simulink model "MGTestSystem_4bus"  (R2021b)
settings: Solver=VariableStepAuto  StartTime=0.0  StopTime=4  RelTol=1e-3
PreLoadFcn:
  | addpath Icons
  | addpath Util
InitFcn:
  | clc
  | %clear all
  | 
  | nDER = 4;
  | xssum = zeros(nDER*2,1);
  | save XSSUM xssum
  | 
  | Ts_Control=1e-4;       % local control time step
  | Ts_Simulation=5e-5;   %simulation time step
  | Ts_Power=5e-5;   % measurement time step
  | Tdisc=0.8;     % time setting for disconnecting from the main grid
  | 
  | Iref = 0.3;  % in p.u.
  | Iqref = 0;  % in p.u.
  | 
  | Ts_secondary =3e-2;   %  secondary control time step
  | %Ts_PMU = 1/60;
  | 
  | ft2km=3.0480e-04;
  | 
  | KPdroop=3.4e-4;
  | KQdroop=1e-3/1;
  | KPdroop2=4.5e-4;
  | KQdroop2=1.5e-3/1;
  | 
  | %KWinvdroop = 20.0;
  | %KVinvdroop = 16.7;
  | %KWinvdroop = 0.05;
  | %KVinvdroop = 0.08;
  | 
  | KWinvdroop = 1/(2*pi*KPdroop);
  | KVinvdroop = 1/(2*pi*KQdroop)
  | KWinvdroop2 = 1/(2*pi*KPdroop2);
  | KVinvdroop2 = 1/(2*pi*KQdroop2)
  | %KVinvdroop = 1/(KQdroop);
  | %KVinvdroop2 = 1/(KQdroop2);
  | %KWinvdroop = 1/(KPdroop);
  | %KWinvdroop2 = 1/(KPdroop2);
  | 
  | droopv1=1/KVinvdroop
  | droopv2=1/KVinvdroop2
  | 
  | 
  | 
  | 
  | wfilter = 35;
  | Rv=0.0;
  | Lv=0e-3;
  | 
  | div=1;
  | 
  | 
  | Kpac=0.1/1;
  | Kiac=420/1;
  | Kpaci=15/div;
  | Kiaci=2e3/div;
  | Kpac2=0.05/1;
  | Kiac2=390/1;
  | Kpaci2=15/div;
  | Kiaci2=1.6e3/div;
  | 
  | 
  | Kpac=0.5/div;
  | Kiac=53/div;
  | Kpaci=45/div;
  | Kiaci=450/div;
  | Kpac2=0.5/div;
  | Kiac2=34/div;
  | Kpaci2=35/div;
  | Kiaci2=353/div;
  | 
  | 
  | Kpac=0.1256/div;
  | Kiac=950/div;
  | Kpaci=20.6/div;
  | Kiaci=1522.7/div;
  | Kpac2=0.1256/div;
  | Kiac2=591/div;
  | Kpaci2=20.6/div;
  | Kiaci2=1522.7/div;
  | 
  | 
  | Kpac=0.5;  % K_I for voltage PI
  | Kiac=523;  % K_I for voltage PI
  | Kpac2=0.5; % K_P for voltage PI 2
  | Kiac2=523; % K_I for voltage PI 2
  | Kpaci=0.3;  % K_P for current PI
  | Kiaci=635;   % K_I for current PI
  | Kpaci2=0.3;  % K_P for current PI 2
  | Kiaci2=635;  % K_I for current PI 2
  | 
  | 
  | k=1;
  | 
  | Pvscr = 30e3;
  | VDC = 950;
  | 
  | %PDERS1 = 12e3;
  | %QDERS1 = 6e3;
  | %PDERS2 = 12e3;
  | %QDERS2 = 6e3;
  | %PDERS3 = 12e3;
  | %QDERS3 = 6e3;
  | %PDERS4 = 12e3;
  | %QDERS4= 6e3;
  | 
  | %[params,indctor] = initfuncv1();
undefined symbols (not defined in the file or in its folder): D1, Delta, Ion, Lithium
libraries: spsStairGeneratorLib x24, spsThreePhaseSeriesRLCBranchLib x24, powerlib_extras x23, spsSeriesRLCBranchLib x20, spsThreePhaseVIMeasurementLib x18, slpidlib x18, spsThreePhaseBreakerLib x15, spsRMSLib x10, spsThreePhaseSeriesRLCLoadLib x8, spsVoltageMeasurementLib x8, spsPMUPLLBasedPositiveSequenceLib x6, spsPowerLib x5
(part 1 of 7)
settings Model: Creator=gongx  LastModifiedBy=gongx
settings SolverCC: ZeroCrossAlgorithm=Adaptive
settings DataIOCC: SaveOutput=off  SignalLogging=off  DSMLogging=off  ReturnWorkspaceOutputs=off
settings DebuggingCC: MaskedZcDiagnostic=none  IgnoredZcDiagnostic=none  UnderSpecifiedDimensionMsg=warning

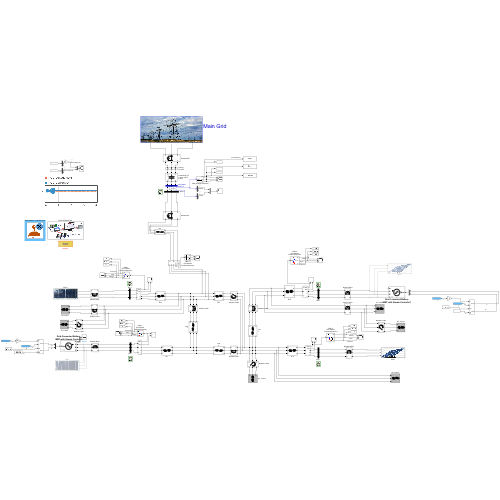
[thumbnail: Simulink's stored preview of the top-level diagram]
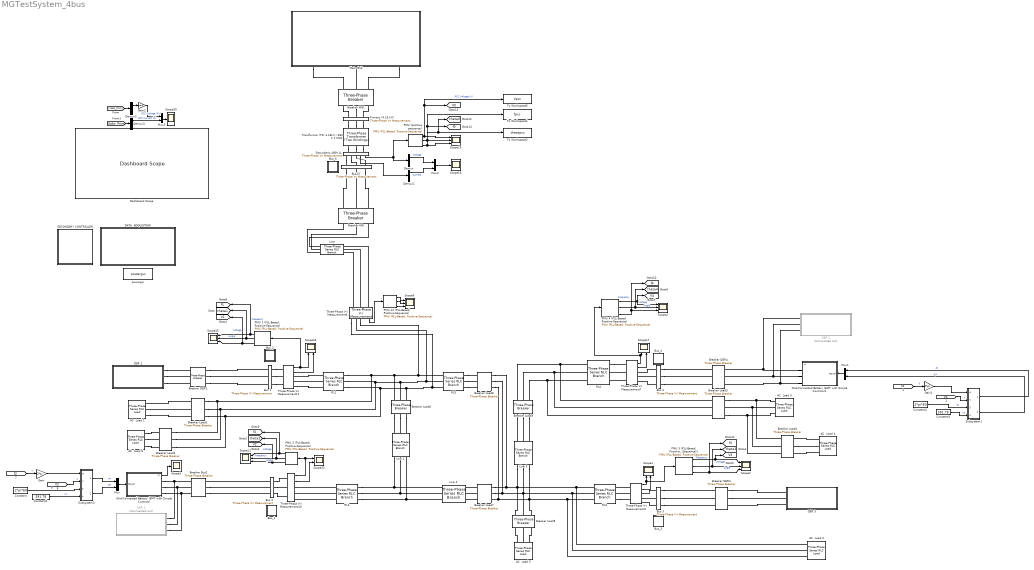
== system MGTestSystem_4bus ==
  " Bus13" : spsThreePhaseVIMeasurementLib/Three-Phase V-I Measurement  VoltageMeasurement=phase-to-ground  SetLabelV=on  LabelV=Vabc_LL_Bus13  Vpu=off  VpuLL=off  CurrentMeasurement=yes  SetLabelI=on  LabelI=Iabc_LL_Bus13  Ipu=off  Pbase=100e6  Vbase=500e3  OutputType=Complex  PhasorSimulation=off  PSBequivalent=0
  AC  Load 1 : spsThreePhaseSeriesRLCLoadLib/Three-Phase Series RLC Load  LConnTagsString=A|B|C  Configuration=Y (grounded)  NominalVoltage=480  Vabc=[1e3 1e3 1e3]  Vabcp=[1e3 1e3 1e3]  NominalFrequency=60  UnbalancedPower=off  ActivePower=20e3  InductivePower=9e3  CapacitivePower=0  Pabc=[10e3 9e3 11e3]  QLabc=[100 90 110]  QCabc=[100 90 110]  Pabcp=[10e3 9e3 11e3]  QLabcp=[100 90 110]  QCabcp=[100 90 110]  Measurements=None  LoadType=constant PQ
  AC  Load 2 : spsThreePhaseSeriesRLCLoadLib/Three-Phase Series RLC Load  LConnTagsString=A|B|C  Configuration=Y (grounded)  NominalVoltage=480  Vabc=[1e3 1e3 1e3]  Vabcp=[1e3 1e3 1e3]  NominalFrequency=60  UnbalancedPower=off  ActivePower=16e3  InductivePower=9e3  CapacitivePower=0  Pabc=[10e3 9e3 11e3]  QLabc=[100 90 110]  QCabc=[100 90 110]  Pabcp=[10e3 9e3 11e3]  QLabcp=[100 90 110]  QCabcp=[100 90 110]  Measurements=None  LoadType=constant PQ
  AC  Load 3 : spsThreePhaseSeriesRLCLoadLib/Three-Phase Series RLC Load  LConnTagsString=A|B|C  Configuration=Y (grounded)  NominalVoltage=480  Vabc=[1e3 1e3 1e3]  Vabcp=[1e3 1e3 1e3]  NominalFrequency=60  UnbalancedPower=off  ActivePower=12e3  InductivePower=6e3  CapacitivePower=0  Pabc=[10e3 9e3 11e3]  QLabc=[100 90 110]  QCabc=[100 90 110]  Pabcp=[10e3 9e3 11e3]  QLabcp=[100 90 110]  QCabcp=[100 90 110]  Measurements=None  LoadType=constant PQ
  AC  Load 4 : spsThreePhaseSeriesRLCLoadLib/Three-Phase Series RLC Load  LConnTagsString=A|B|C  Configuration=Y (grounded)  NominalVoltage=480  Vabc=[1e3 1e3 1e3]  Vabcp=[1e3 1e3 1e3]  NominalFrequency=60  UnbalancedPower=off  ActivePower=10e3  InductivePower=6e3  CapacitivePower=0  Pabc=[10e3 9e3 11e3]  QLabc=[100 90 110]  QCabc=[100 90 110]  Pabcp=[10e3 9e3 11e3]  QLabcp=[100 90 110]  QCabcp=[100 90 110]  Measurements=None  LoadType=constant PQ
  AC  Load 5 : spsThreePhaseSeriesRLCLoadLib/Three-Phase Series RLC Load  LConnTagsString=A|B|C  Configuration=Y (grounded)  NominalVoltage=480  Vabc=[1e3 1e3 1e3]  Vabcp=[1e3 1e3 1e3]  NominalFrequency=60  UnbalancedPower=off  ActivePower=60e3  InductivePower=30e3  CapacitivePower=0  Pabc=[10e3 9e3 11e3]  QLabc=[100 90 110]  QCabc=[100 90 110]  Pabcp=[10e3 9e3 11e3]  QLabcp=[100 90 110]  QCabcp=[100 90 110]  Measurements=None  LoadType=constant PQ
  AC  Load 6 : spsThreePhaseSeriesRLCLoadLib/Three-Phase Series RLC Load  LConnTagsString=A|B|C  Configuration=Y (grounded)  NominalVoltage=480  Vabc=[1e3 1e3 1e3]  Vabcp=[1e3 1e3 1e3]  NominalFrequency=60  UnbalancedPower=off  ActivePower=50e3  InductivePower=30e3  CapacitivePower=0  Pabc=[10e3 9e3 11e3]  QLabc=[100 90 110]  QCabc=[100 90 110]  Pabcp=[10e3 9e3 11e3]  QLabcp=[100 90 110]  QCabcp=[100 90 110]  Measurements=None  LoadType=constant PQ
  "Breaker Bus2 " : spsThreePhaseBreakerLib/Three-Phase Breaker  InitialState=closed  SwitchA=on  SwitchB=on  SwitchC=on  SwitchTimes=[113.3 200]  External=off  BreakerResistance=0.001  SnubberResistance=1e6  SnubberCapacitance=inf  Measurements=None
  Breaker DER1 : spsThreePhaseBreakerLib/Three-Phase Breaker  InitialState=closed  SwitchA=on  SwitchB=on  SwitchC=on  SwitchTimes="[10.9  314]"  External=off  BreakerResistance=0.001  SnubberResistance=1e6  SnubberCapacitance=inf  Measurements=None
  Breaker DER3 : spsThreePhaseBreakerLib/Three-Phase Breaker  InitialState=closed  SwitchA=on  SwitchB=on  SwitchC=on  SwitchTimes="[112.7  123.4]"  External=off  BreakerResistance=0.001  SnubberResistance=1e6  SnubberCapacitance=inf  Measurements=None
  Breaker DER4 : spsThreePhaseBreakerLib/Three-Phase Breaker  InitialState=closed  SwitchA=on  SwitchB=on  SwitchC=on  SwitchTimes="[112.7  300.4]"  External=off  BreakerResistance=0.001  SnubberResistance=1e6  SnubberCapacitance=inf  Measurements=None
  Breaker Load1 : spsThreePhaseBreakerLib/Three-Phase Breaker  InitialState=closed  SwitchA=on  SwitchB=on  SwitchC=on  SwitchTimes="[111.8  113.3]"  External=off  BreakerResistance=0.001  SnubberResistance=1e6  SnubberCapacitance=inf  Measurements=None
  Breaker Load2 : spsThreePhaseBreakerLib/Three-Phase Breaker  InitialState=open  SwitchA=on  SwitchB=on  SwitchC=on  SwitchTimes="[10.9  112.3]"  External=off  BreakerResistance=0.001  SnubberResistance=1e6  SnubberCapacitance=inf  Measurements=None
  Breaker Load3 : spsThreePhaseBreakerLib/Three-Phase Breaker  InitialState=closed  SwitchA=on  SwitchB=on  SwitchC=on  SwitchTimes="[112.2  113.3]"  External=off  BreakerResistance=0.001  SnubberResistance=1e6  SnubberCapacitance=inf  Measurements=None
  Breaker Load4 : spsThreePhaseBreakerLib/Three-Phase Breaker  InitialState=open  SwitchA=on  SwitchB=on  SwitchC=on  SwitchTimes="[13.0  120.6]"  External=off  BreakerResistance=0.001  SnubberResistance=1e6  SnubberCapacitance=inf  Measurements=None
  Breaker Load5 : spsThreePhaseBreakerLib/Three-Phase Breaker  InitialState=open  SwitchA=on  SwitchB=on  SwitchC=on  SwitchTimes="[11.5  212.3]"  External=off  BreakerResistance=0.001  SnubberResistance=1e6  SnubberCapacitance=inf  Measurements=None
  Breaker Load6 : spsThreePhaseBreakerLib/Three-Phase Breaker  InitialState=closed  SwitchA=on  SwitchB=on  SwitchC=on  SwitchTimes="[111.5  112]"  External=off  BreakerResistance=0.001  SnubberResistance=1e6  SnubberCapacitance=inf  Measurements=None
  Breaker Load7 : spsThreePhaseBreakerLib/Three-Phase Breaker  InitialState=closed  SwitchA=on  SwitchB=on  SwitchC=on  SwitchTimes="[12.5  112]"  External=off  BreakerResistance=0.001  SnubberResistance=1e6  SnubberCapacitance=inf  Measurements=None
  Breaker Load8 : spsThreePhaseBreakerLib/Three-Phase Breaker  InitialState=open  SwitchA=on  SwitchB=on  SwitchC=on  SwitchTimes="[11.5  112]"  External=off  BreakerResistance=0.001  SnubberResistance=1e6  SnubberCapacitance=inf  Measurements=None
  Breaker Load9 : spsThreePhaseBreakerLib/Three-Phase Breaker  InitialState=closed  SwitchA=on  SwitchB=on  SwitchC=on  SwitchTimes="[11.0  112]"  External=off  BreakerResistance=0.001  SnubberResistance=1e6  SnubberCapacitance=inf  Measurements=None
  Breaker MG : spsThreePhaseBreakerLib/Three-Phase Breaker  InitialState=closed  SwitchA=on  SwitchB=on  SwitchC=on  SwitchTimes=Tdisc-0.1  External=off  BreakerResistance=0.001  SnubberResistance=1e6  SnubberCapacitance=inf  Measurements=None
  Breaker MG1 : spsThreePhaseBreakerLib/Three-Phase Breaker  InitialState=closed  SwitchA=on  SwitchB=on  SwitchC=on  SwitchTimes=11  External=off  BreakerResistance=0.001  SnubberResistance=1e6  SnubberCapacitance=inf  Measurements=None
  Bus 1 : spsThreePhaseVIMeasurementLib/Three-Phase V-I Measurement  VoltageMeasurement=phase-to-ground  SetLabelV=on  LabelV=Vabc_LL_Bus1  Vpu=off  VpuLL=off  CurrentMeasurement=yes  SetLabelI=on  LabelI=Iabc_LL_Bus1  Ipu=off  Pbase=100e6  Vbase=380/sqrt(2)  OutputType=Complex  PhasorSimulation=off  PSBequivalent=0
  Bus 2 : spsThreePhaseVIMeasurementLib/Three-Phase V-I Measurement  VoltageMeasurement=phase-to-ground  SetLabelV=on  LabelV=Vabc_LL_Bus2  Vpu=off  VpuLL=off  CurrentMeasurement=yes  SetLabelI=on  LabelI=Iabc_LL_Bus2  Ipu=off  Pbase=100e6  Vbase=25e3  OutputType=Complex  PhasorSimulation=off  PSBequivalent=0
  Bus 3 : spsThreePhaseVIMeasurementLib/Three-Phase V-I Measurement  VoltageMeasurement=phase-to-ground  SetLabelV=on  LabelV=Vabc_LL_Bus3  Vpu=off  VpuLL=off  CurrentMeasurement=yes  SetLabelI=on  LabelI=Iabc_LL_Bus3  Ipu=off  Pbase=100e6  Vbase=380/sqrt(2)  OutputType=Complex  PhasorSimulation=off  PSBequivalent=0
  Bus 4 : spsThreePhaseVIMeasurementLib/Three-Phase V-I Measurement  VoltageMeasurement=phase-to-ground  SetLabelV=on  LabelV=Vabc_LL_Bus4  Vpu=off  VpuLL=off  CurrentMeasurement=yes  SetLabelI=on  LabelI=Iabc_LL_Bus4  Ipu=off  Pbase=100e6  Vbase=380/sqrt(2)  OutputType=Complex  PhasorSimulation=off  PSBequivalent=0
  Bus_1 : Subsystem
      mask Display: image('Icons\S_meeter.png');
  Bus_2 : Subsystem
      mask Display: image('Icons\S_meeter.png');
  Bus_3 : Subsystem
      mask Display: image('Icons\S_meeter.png');
  Bus_4 : Subsystem
      mask Display: image('Icons\S_meeter.png');
  Bus_6 : Subsystem
      mask Display: image('Icons\S_meeter.png');
  Constant : Constant  Value=2*pi*60
  Constant1 : Constant  Value=391.78
  Constant2 : Constant  Value=2*pi*60
  Constant3 : Constant  Value=391.78
  DATA  ADQUISITION : Subsystem
      mask Display: image('Icons\SCADA.png');
  DER 1 : Subsystem
      mask Display: image('$imagefile'); % Use "Edit Image" on toolstrip to change.
  DER 2 : Subsystem  Commented=on
      mask Display: image('$imagefile'); % Use "Edit Image" on toolstrip to change.
  DER 3 : Subsystem
      mask Display: image('$imagefile'); % Use "Edit Image" on toolstrip to change.
  DER 4 : Subsystem  Commented=on
      mask Display: image('$imagefile'); % Use "Edit Image" on toolstrip to change.
  Dashboard Scope : DashboardScope
  Demux{,1..3} (4 alike) : Demux  Outputs=3
  Gain : Gain  Gain=2*pi
  Gain1 : Gain  Gain=2*pi
  Gain2 : Gain  Gain=1e-3
  Grid-Connected Battery (EMT with Simple Controls) : Subsystem  AncestorBlock=|  mask{Pmod=1, Vnom_dc=960, Bcap=100, Vnom_prim=480, Fnom=60, Ts=Ts_Simulation, Ts_Control=Ts_Control}
      | Library_DERs_in_Microgrid/Grid-Connected Battery
      | (EMT with Simple Controls)
      mask prompts: Pmod "Scale Battery, Multiplier for 100 kW"; Vnom_dc "Nominal Battery Voltage, V"; Bcap "Battery Capacity, Ah"; Vnom_prim "Nominal Grid Connection L-L Voltage, Vrms"; Fnom "Grid Frequency, Fnom [Hz]"; Ts "Simulation Time Step, Ts [s]"; Ts_Control "Controller Time Step, Ts_Control"
      mask init:
      | Pnom = Pmod*100e3;      % Inverter nominal 3-phase power (VA)
      | Vnom_dc = 480;     % Nominal DC link voltage (V)
      | % Vnom_prim = 25e3;  % Nominal inverter primary line-to-line voltage(Vrms)
      | Vnom_sec= 0.85*Vnom_dc/2/sqrt(2)*sqrt(3); % Nominal inverter secondary line-to-line voltage (Vrms)
      | 
      | TotalLeakage = 0.06;   % Transformer total leakage (pu)
      | Rxf = TotalLeakage/25;
      | Lxf = TotalLeakage;
      | 
      | % Inverter choke RL [Rpu Lpu]
      | Rchoke = 0.15/100;
      | Lchoke = 0.15;
      | Zbase = Vnom_sec^2/Pnom;
      | 
      | % Filter C Parameters
      | Qc = 0.1*Pnom;     % Capacitive reactive power (var)
      | Pc = Qc/50;        % Active power (W)      
      | 
      | Clink = 2 * 3/4 * (Pnom/Fnom*2/Vnom_dc^2); % DC link energy for 3/4 cycle of Pnom
      | 
      | % VDC regulator (VDCreg)
      | Kp_VDCreg = 2;           % Proportional gain
      | Ki_VDCreg = 400;        % Integral gain
      | 
      | Rtot_pu = Rxf + Rchoke; % Feedforward values
      | Ltot_pu = Lxf + Lchoke; % Feedforward values
      | 
      | Kp_Ireg = 0.3;          % Proportional gain
      | Ki_Ireg = 20;           % Integral gain
      mask Display: plot(-80,-50,80,50,[0,9,18,24,29,30,29,24,18,9,0,-9,-18,-24,-29,-30,-29,-24,-18,-9,0],[30,29,24,18,9,0,-9,-18,-24,-29,-30,-29,-24,-18,-9,0,9,18,24,29,30],[-50],[0],[50],[0],[45 35 40 40 40],[15 15 15 20 10],[1 2 3 4 5 6 7 8 9 10 11 12 13 14 15 16 17 18 19 20 21].*1.5-15,[0,9,18,24,29,30,29,24,18,9,0,-9,-18,-24,-29,-30,-29,-24,-18,-9,0]./2.4)
  Grid-Connected Battery (EMT with Simple Controls)1 : Subsystem  AncestorBlock=|  mask{Pmod=1, Vnom_dc=960, Bcap=100, Vnom_prim=480, Fnom=60, Ts=Ts_Simulation, Ts_Control=Ts_Control}
      | Library_DERs_in_Microgrid/Grid-Connected Battery
      | (EMT with Simple Controls)
      mask prompts: Pmod "Scale Battery, Multiplier for 100 kW"; Vnom_dc "Nominal Battery Voltage, V"; Bcap "Battery Capacity, Ah"; Vnom_prim "Nominal Grid Connection L-L Voltage, Vrms"; Fnom "Grid Frequency, Fnom [Hz]"; Ts "Simulation Time Step, Ts [s]"; Ts_Control "Controller Time Step, Ts_Control"
      mask init: same as MGTestSystem_4bus/Grid-Connected Battery (EMT with Simple Controls)
      mask Display: plot(-80,-50,80,50,[0,9,18,24,29,30,29,24,18,9,0,-9,-18,-24,-29,-30,-29,-24,-18,-9,0],[30,29,24,18,9,0,-9,-18,-24,-29,-30,-29,-24,-18,-9,0,9,18,24,29,30],[-50],[0],[50],[0],[45 35 40 40 40],[15 15 15 20 10],[1 2 3 4 5 6 7 8 9 10 11 12 13 14 15 16 17 18 19 20 21].*1.5-15,[0,9,18,24,29,30,29,24,18,9,0,-9,-18,-24,-29,-30,-29,-24,-18,-9,0]./2.4)
  Line : spsThreePhaseSeriesRLCBranchLib/Three-Phase Series RLC Branch  LConnTagsString=A|B|C  RConnTagsString=A|B|C  BranchType=RL  Resistance=0.08  Inductance=0.1e-3  Capacitance=1e-6  Measurements=None
  Line 1 : spsThreePhaseSeriesRLCBranchLib/Three-Phase Series RLC Branch  LConnTagsString=A|B|C  RConnTagsString=A|B|C  BranchType=RL  Resistance=0.15  Inductance=0.42e-3  Capacitance=1e-6  Measurements=None
  Line 2 : spsThreePhaseSeriesRLCBranchLib/Three-Phase Series RLC Branch  LConnTagsString=A|B|C  RConnTagsString=A|B|C  BranchType=RL  Resistance=0.35  Inductance=0.33e-3  Capacitance=1e-6  Measurements=None
  Line 3 : spsThreePhaseSeriesRLCBranchLib/Three-Phase Series RLC Branch  LConnTagsString=A|B|C  RConnTagsString=A|B|C  BranchType=RL  Resistance=0.23  Inductance=0.55e-3  Capacitance=1e-6  Measurements=None
  "Main Grid " : Subsystem
      mask Display: image('$imagefile'); % Use "Edit Image" on toolstrip to change.
  Mux{,1..3} (4 alike) : Mux  Inputs=2
  "PMU (positive sequence) " : spsPMUPLLBasedPositiveSequenceLib/PMU (PLL-Based, Positive-Sequence)  nominalFrequency=60  samplingRate=64  reportingFactor=1
      settings: SourceProductBaseCode=PS
  "PMU 1 (PLL-Based, Positive-Sequence)" : spsPMUPLLBasedPositiveSequenceLib/PMU (PLL-Based, Positive-Sequence)  nominalFrequency=60  samplingRate=64  reportingFactor=1
      settings: SourceProductBaseCode=PS
  "PMU 12 (PLL-Based, Positive-Sequence)" : spsPMUPLLBasedPositiveSequenceLib/PMU (PLL-Based, Positive-Sequence)  nominalFrequency=60  samplingRate=64  reportingFactor=1
      settings: SourceProductBaseCode=PS
  "PMU 2 (PLL-Based, Positive-Sequence)" : spsPMUPLLBasedPositiveSequenceLib/PMU (PLL-Based, Positive-Sequence)  nominalFrequency=60  samplingRate=64  reportingFactor=1
      settings: SourceProductBaseCode=PS
  "PMU 3 (PLL-Based, Positive-Sequence)1" : spsPMUPLLBasedPositiveSequenceLib/PMU (PLL-Based, Positive-Sequence)  nominalFrequency=60  samplingRate=64  reportingFactor=1
      settings: SourceProductBaseCode=PS
  "PMU 4 (PLL-Based, Positive-Sequence)" : spsPMUPLLBasedPositiveSequenceLib/PMU (PLL-Based, Positive-Sequence)  nominalFrequency=60  samplingRate=64  reportingFactor=1
      settings: SourceProductBaseCode=PS
  Primary (4.16 kV) : spsThreePhaseVIMeasurementLib/Three-Phase V-I Measurement  VoltageMeasurement=phase-to-ground  SetLabelV=on  LabelV=Vabc_Prim  Vpu=off  VpuLL=on  CurrentMeasurement=yes  SetLabelI=on  LabelI=Iabc_Prim  Ipu=off  Pbase=100e6  Vbase=4.16e3/sqrt(2)  OutputType=Magnitude  PhasorSimulation=off  PSBequivalent=0
  RL1 : spsThreePhaseSeriesRLCBranchLib/Three-Phase Series RLC Branch  LConnTagsString=A|B|C  RConnTagsString=A|B|C  BranchType=RL  Resistance=0.08  Inductance=0.35e-3  Capacitance=1e-9  Measurements=None
  RL2 : spsThreePhaseSeriesRLCBranchLib/Three-Phase Series RLC Branch  LConnTagsString=A|B|C  RConnTagsString=A|B|C  BranchType=RL  Resistance=0.08  Inductance=0.35e-3  Capacitance=1e-9  Measurements=None
  RL3 : spsThreePhaseSeriesRLCBranchLib/Three-Phase Series RLC Branch  LConnTagsString=A|B|C  RConnTagsString=A|B|C  BranchType=RL  Resistance=0.09  Inductance=0.45e-3  Capacitance=1e-9  Measurements=None
  RL4 : spsThreePhaseSeriesRLCBranchLib/Three-Phase Series RLC Branch  LConnTagsString=A|B|C  RConnTagsString=A|B|C  BranchType=RL  Resistance=0.09  Inductance=0.45e-3  Capacitance=1e-9  Measurements=None
  RL5 : spsThreePhaseSeriesRLCBranchLib/Three-Phase Series RLC Branch  LConnTagsString=A|B|C  RConnTagsString=A|B|C  BranchType=RL  Resistance=0.08  Inductance=0.35e-3  Capacitance=1e-9  Measurements=None
  SECONDARY CONTROLLER : Subsystem
      mask Display: image('$imagefile'); % Use "Edit Image" on toolstrip to change.
  Scope{1,17,23..24} (4 alike) : Scope  NumInputPorts=2
  Scope{2,4,6,11,15,25} (6 alike) : Scope  NumInputPorts=3
  Scope16 : Scope
  Scope3 : Scope
  Scope30 : Scope
  Secundario 480V LL : spsThreePhaseVIMeasurementLib/Three-Phase V-I Measurement  VoltageMeasurement=phase-to-ground  SetLabelV=off  LabelV=Vabc_Sec_pu  Vpu=off  VpuLL=on  CurrentMeasurement=yes  SetLabelI=off  LabelI=Iabc_Sec_pu  Ipu=off  Pbase=250e6  Vbase=480/sqrt(2)  OutputType=Magnitude  PhasorSimulation=off  PSBequivalent=0
  Subsystem1 : Subsystem  mask{Kp=KWinvdroop, Kq=KVinvdroop, F0=0}
      mask prompts: F0 "F0(Hz)"
  Subsystem2 : Subsystem  mask{Kp=KWinvdroop, Kq=KVinvdroop, F0=0}
      mask prompts: F0 "F0(Hz)"
  Three-Phase V-I Measurement{2,7,9..10,12} (5 alike) : spsThreePhaseVIMeasurementLib/Three-Phase V-I Measurement  VoltageMeasurement=phase-to-ground  SetLabelV=off  LabelV=Vabc  Vpu=off  VpuLL=off  CurrentMeasurement=yes  SetLabelI=off  LabelI=Iabc  Ipu=off  Pbase=100e6  Vbase=500e3  OutputType=Complex  PhasorSimulation=off  PSBequivalent=0
  To Workspace1 : ToWorkspace  VariableName=fpcc  SaveFormat=Structure With Time  SampleTime=-1
      settings: Save2DSignal=2-D array (concatenate along first dimension)
  To Workspace2 : ToWorkspace  VariableName=thetapcc  SaveFormat=Structure With Time  SampleTime=-1
      settings: Save2DSignal=2-D array (concatenate along first dimension)
  To Workspace5 : ToWorkspace  VariableName=Vpcc  SaveFormat=Structure With Time  SampleTime=-1
      settings: Save2DSignal=2-D array (concatenate along first dimension)
  Transformer (T3) 4.16kV / 480 V 1 MVA : spsThreePhaseTransformerTwoWindingsLib/Three-Phase Transformer (Two Windings)  Winding1Connection=Yg  Winding2Connection=Yg  CoreType=Three single-phase transformers  SetSaturation=off  Hysteresis=off  DataFile='hysteresis'  SetInitialFlux=off  Measurements=None  UNITS=pu  NominalPower=[5e6 , 60]  Winding1=[4.16e3 , 0.015/2 , 0.015/(2*377)]  Winding2=[480, 0.015/2 , 0.015/(2*377)]  Rm=500  Lm=500  L0=0.5  Saturation="[ 0,0  ;  0.005,1.2  ;  1.0,1.4 ]"  InitialFluxes=[ 0.8 , -0.8 , 0.7 ]  BreakLoop=off  DiscreteSolver=Trapezoidal iterative  DataType=off  TransfoNumber=0
  powergui : spspowerguiLib/powergui  Priority=1  SimulationMode=Discrete  SampleTime=Ts_Simulation  frequency=60  Iterations=50  frequencyindice=0  Pbase=100e6  ErrMax=1e-4  UnitsV=kV  UnitsW=MW  buscounter=0  FunctionMessages=off  echomessages=off  EnableUseOfTLC=off  CurrentSourceSwitches=off  DisableSnubberDevices=off  DisableRonSwitches=off  DisableVfSwitches=off  DisplayEquations=off  AutomaticDiscreteSolvers=off  SolverType=Tustin/Backward Euler (TBE)  Interpol=off  ExternalGateDelay=off  methode=off  Ts=0  x0status=steady  SPID=off  SwTol=0  HookPort=off  NonlinearTolerance=0  nMaxIteration=15  ContinueOnMaxIteration=on  RestoreLinks=warning  ResistiveCurrentMeasurement=off  Frange=[0:2:500]  Ylog=off  Xlog=on  ShowGrid=off  save=off  variable=ZData  structure=0  ZoomFFT=off  StartTime=0.0  cycles=1  DisplayStyle=1  fundamental=60  FreqAxis=off  MaxFrequency=1000  frequencyindicesteady=1  RmsSteady=1  display=off
  tag scope: V0=global, V1=global, V2=global, V3=global, V4=global, f0=global, f1=global, f2=global, f3=global, f4=global, theta0=global, theta1=global, theta2=global, theta3=global, theta4=global
  wires:
  Three-Phase V-I Measurement10/2 -> Scope23/2
  "PMU 1 (PLL-Based, Positive-Sequence)"/1 -> [V1], Scope25/3  "Voltage"
  Three-Phase V-I Measurement12/2 -> Scope24/2
  "PMU 1 (PLL-Based, Positive-Sequence)"/3 -> Scope25/1, [f1]  "Frequency"
  "PMU 2 (PLL-Based, Positive-Sequence)"/3 -> Scope11/1, [f2]  "Frequency"
  Three-Phase V-I Measurement10/1 -> Scope23/1, "PMU 2 (PLL-Based, Positive-Sequence)"/1
  Three-Phase V-I Measurement12/1 -> Scope24/1, "PMU 1 (PLL-Based, Positive-Sequence)"/1
  "PMU 2 (PLL-Based, Positive-Sequence)"/2 -> Scope11/2, [theta2]  "Angle"
  "PMU 1 (PLL-Based, Positive-Sequence)"/2 -> Scope25/2, [theta1]  "Angle"
  "PMU 4 (PLL-Based, Positive-Sequence)"/2 -> [theta4], Scope4/2  "Angle"
  Three-Phase V-I Measurement7/2 -> Scope17/2
  "PMU 4 (PLL-Based, Positive-Sequence)"/3 -> [f4], Scope4/3  "Frequency"
  Three-Phase V-I Measurement7/1 -> "PMU 4 (PLL-Based, Positive-Sequence)"/1, Scope17/1
  "PMU 4 (PLL-Based, Positive-Sequence)"/1 -> Scope4/1, [V4]  "Voltage"
  "PMU 3 (PLL-Based, Positive-Sequence)1"/1 -> [V3], Scope2/1  "Voltage"
  Three-Phase V-I Measurement2/1 -> "PMU 3 (PLL-Based, Positive-Sequence)1"/1, Scope1/1
  "PMU 3 (PLL-Based, Positive-Sequence)1"/3 -> [f3], Scope2/3  "Frequency"
  Three-Phase V-I Measurement2/2 -> Scope1/2
  "PMU 3 (PLL-Based, Positive-Sequence)1"/2 -> [theta3], Scope2/2  "Angle"
  "PMU 2 (PLL-Based, Positive-Sequence)"/1 -> [V2], Scope11/3  "Voltage"
  Subsystem2/2(Qref) -> Mux/2  "Q*"
  Subsystem2/1(Pref) -> Mux/1  "P*"
  Mux/1 -> Grid-Connected Battery (EMT with Simple Controls)/1(PQref)
  Mux1/1 -> Grid-Connected Battery (EMT with Simple Controls)1/1(PQref)
  Grid-Connected Battery (EMT with Simple Controls)/1(m) -> Scope3/1
  Constant/1 -> Subsystem2/3(w0)  "f*"
  [V2] -> Subsystem2/2(V)  "V"
  [f2] -> Gain/1  "f"
  Gain/1 -> Subsystem2/1(w)
  Subsystem1/1(Pref) -> Mux1/1  "P*"
  [f4] -> Gain1/1  "f"
  Constant2/1 -> Subsystem1/3(w0)  "f*"
  [V4] -> Subsystem1/2(V)  "V"
  Constant3/1 -> Subsystem1/4(V0)  "V*"
  Subsystem1/2(Qref) -> Mux1/2  "Q*"
  Gain1/1 -> Subsystem1/1(w)
  "PMU 12 (PLL-Based, Positive-Sequence)"/3 -> Scope6/3
  "PMU 12 (PLL-Based, Positive-Sequence)"/1 -> Scope6/1
  Three-Phase V-I Measurement9/1 -> "PMU 12 (PLL-Based, Positive-Sequence)"/1
  Demux/1 -> Mux2/1  "Voltage"
  Secundario 480V LL/1 -> "PMU (positive sequence) "/1, Demux/1
  Secundario 480V LL/2 -> Demux1/1
  Gain2/1 -> Mux3/1  "PCC Voltage (kV)"
  Demux1/1 -> Mux2/2  "Current"
  [Vabc_Prim] -> Demux2/1
  "PMU 12 (PLL-Based, Positive-Sequence)"/2 -> Scope6/2
  Demux2/1 -> Gain2/1
  Mux3/1 -> Scope30/1
  Demux3/1 -> Mux3/2  "PCC Current (A)"
  Mux2/1 -> Scope16/1
  [Iabc_Prim] -> Demux3/1
  Constant1/1 -> Subsystem2/4(V0)  "V*"
  "PMU (positive sequence) "/2 -> [theta0], To Workspace2/1, Scope15/2
  "PMU (positive sequence) "/1 -> [V0], To Workspace5/1, Scope15/1  "PCC Voltage (V)"
  "PMU (positive sequence) "/3 -> To Workspace1/1, [f0], Scope15/3
  connections:
  Line 2/RConn3 -- Line 1/RConn3 -- RL2/RConn3
  Line 1/RConn2 -- Line 2/RConn2 -- RL2/RConn2
  Bus 2/RConn3 -- Three-Phase V-I Measurement10/LConn3
  Bus 1/RConn3 -- Three-Phase V-I Measurement12/LConn1
  Bus 1/RConn1 -- Three-Phase V-I Measurement12/LConn3
  "Breaker Bus2 "/RConn2 -- Bus 2/LConn2
  Bus 2/RConn2 -- Three-Phase V-I Measurement10/LConn2
  Bus 1/RConn2 -- Three-Phase V-I Measurement12/LConn2
  Bus 2/RConn1 -- Three-Phase V-I Measurement10/LConn1
  "Breaker Bus2 "/RConn1 -- Bus 2/LConn3
  Bus 4/LConn2 -- Breaker DER4/LConn2
  Bus 4/LConn1 -- Breaker DER4/LConn3
  Bus 4/RConn2 -- Three-Phase V-I Measurement7/RConn2
  Bus 4/RConn3 -- Three-Phase V-I Measurement7/RConn3
  Bus 4/RConn1 -- Three-Phase V-I Measurement7/RConn1
  Bus 3/LConn3 -- Breaker DER3/LConn1
  Bus 3/RConn2 -- Three-Phase V-I Measurement2/RConn2
  Bus 3/RConn1 -- Three-Phase V-I Measurement2/RConn1
  Bus 3/RConn3 -- Three-Phase V-I Measurement2/RConn3
  Breaker Load3/LConn3 -- Breaker Load9/LConn1 -- RL4/LConn1
  Breaker Load3/LConn2 -- Breaker Load9/LConn2 -- RL4/LConn2
  Breaker Load3/LConn1 -- Breaker Load9/LConn3 -- RL4/LConn3
  DER 1/LConn1 -- Breaker DER1/RConn1
  DER 1/LConn2 -- Breaker DER1/RConn2
  DER 1/LConn3 -- Breaker DER1/RConn3
  Bus 3/LConn1 -- Breaker DER3/LConn3
  Grid-Connected Battery (EMT with Simple Controls)1/RConn1 -- Breaker DER4/RConn3 -- DER 4/LConn1
  Grid-Connected Battery (EMT with Simple Controls)1/RConn2 -- DER 4/LConn2 -- Breaker DER4/RConn2
  Grid-Connected Battery (EMT with Simple Controls)1/RConn3 -- DER 4/LConn3 -- Breaker DER4/RConn1
  Breaker DER3/RConn2 -- DER 3/LConn2
  Breaker DER3/RConn3 -- DER 3/LConn1
  DER 3/LConn3 -- Breaker DER3/RConn1
  Bus 4/LConn3 -- Breaker DER4/LConn1
  Bus 3/LConn2 -- Breaker DER3/LConn2
  Breaker Load3/RConn3 -- Breaker Load4/LConn3 -- AC  Load 3/LConn1
  AC  Load 3/LConn2 -- Breaker Load4/LConn2 -- Breaker Load3/RConn2
  Breaker Load3/RConn1 -- Breaker Load4/LConn1 -- AC  Load 3/LConn3
  AC  Load 5/LConn1 -- Breaker Load5/RConn1
  AC  Load 5/LConn2 -- Breaker Load5/RConn2
  AC  Load 5/LConn3 -- Breaker Load5/RConn3
  Breaker DER1/LConn2 -- Bus 1/LConn2
  Breaker DER1/LConn3 -- Bus 1/LConn1
  Breaker DER1/LConn1 -- Bus 1/LConn3
  Grid-Connected Battery (EMT with Simple Controls)/RConn2 -- DER 2/LConn2 -- "Breaker Bus2 "/LConn2
  Grid-Connected Battery (EMT with Simple Controls)/RConn1 -- DER 2/LConn1 -- "Breaker Bus2 "/LConn3
  Grid-Connected Battery (EMT with Simple Controls)/RConn3 -- DER 2/LConn3 -- "Breaker Bus2 "/LConn1
  Bus 2/LConn1 -- "Breaker Bus2 "/RConn3
  Three-Phase V-I Measurement9/RConn2 -- Breaker Load2/LConn2 -- Breaker Load1/LConn2 -- RL1/RConn2 -- Breaker Load6/LConn2 -- RL5/LConn2
  Three-Phase V-I Measurement9/RConn3 -- Breaker Load2/LConn3 -- Breaker Load1/LConn3 -- RL1/RConn3 -- Breaker Load6/LConn3 -- RL5/LConn3
  Line 1/RConn1 -- Line 2/RConn1 -- RL2/RConn1
  Line 3/RConn3 -- Breaker Load8/LConn3 -- Breaker Load7/LConn3 -- RL3/LConn3 -- AC  Load 2/LConn3 -- Breaker Load5/LConn3
  Line 3/RConn2 -- Breaker Load7/LConn2 -- Breaker Load8/LConn2 -- RL3/LConn2 -- AC  Load 2/LConn2 -- Breaker Load5/LConn2
  Breaker Load1/RConn1 -- AC  Load 1/LConn1
  Breaker Load1/RConn2 -- AC  Load 1/LConn2
  AC  Load 1/LConn3 -- Breaker Load1/RConn3
  AC  Load 6/LConn2 -- Breaker Load2/RConn2
  AC  Load 6/LConn1 -- Breaker Load2/RConn1
  AC  Load 6/LConn3 -- Breaker Load2/RConn3
  Three-Phase V-I Measurement9/RConn1 -- RL5/LConn1 -- Breaker Load2/LConn1 -- Breaker Load1/LConn1 -- RL1/RConn1 -- Breaker Load6/LConn1
  AC  Load 4/LConn1 -- Breaker Load4/RConn3
  Breaker Load4/RConn2 -- AC  Load 4/LConn2
  AC  Load 4/LConn3 -- Breaker Load4/RConn1
  Line 3/RConn1 -- Breaker Load7/LConn1 -- Breaker Load8/LConn1 -- Breaker Load5/LConn1 -- RL3/LConn1 -- AC  Load 2/LConn1
  RL1/LConn2 -- Three-Phase V-I Measurement12/RConn2
  RL1/LConn1 -- Three-Phase V-I Measurement12/RConn1
  Three-Phase V-I Measurement12/RConn3 -- RL1/LConn3
  RL2/LConn1 -- Three-Phase V-I Measurement10/RConn1
  RL2/LConn2 -- Three-Phase V-I Measurement10/RConn2
  RL2/LConn3 -- Three-Phase V-I Measurement10/RConn3
  Three-Phase V-I Measurement2/LConn1 -- RL3/RConn1
  Three-Phase V-I Measurement2/LConn2 -- RL3/RConn2
  RL3/RConn3 -- Three-Phase V-I Measurement2/LConn3
  RL4/RConn1 -- Three-Phase V-I Measurement7/LConn1
  Three-Phase V-I Measurement7/LConn2 -- RL4/RConn2
  Three-Phase V-I Measurement7/LConn3 -- RL4/RConn3
  Breaker Load7/RConn1 -- Line 2/LConn1
  Breaker Load7/RConn2 -- Line 2/LConn2
  Breaker Load7/RConn3 -- Line 2/LConn3
  Breaker Load6/RConn1 -- Line 1/LConn1
  Breaker Load6/RConn2 -- Line 1/LConn2
  Breaker Load6/RConn3 -- Line 1/LConn3
  RL5/RConn2 -- Breaker Load8/RConn2
  RL5/RConn1 -- Breaker Load8/RConn1
  RL5/RConn3 -- Breaker Load8/RConn3
  Breaker Load9/RConn1 -- Line 3/LConn1
  Breaker Load9/RConn2 -- Line 3/LConn2
  Breaker Load9/RConn3 -- Line 3/LConn3
  Primary (4.16 kV)/RConn2 -- Transformer (T3) 4.16kV / 480 V 1 MVA/LConn2
  Line/RConn1 -- Breaker MG/RConn1
  Line/RConn2 -- Breaker MG/RConn2
  Transformer (T3) 4.16kV / 480 V 1 MVA/RConn1 -- Secundario 480V LL/LConn1
  " Bus13"/LConn1 -- Secundario 480V LL/RConn1
  Transformer (T3) 4.16kV / 480 V 1 MVA/RConn2 -- Secundario 480V LL/LConn2
  " Bus13"/RConn3 -- Breaker MG/LConn3
  Secundario 480V LL/RConn3 -- " Bus13"/LConn3
  " Bus13"/RConn2 -- Breaker MG/LConn2
  Three-Phase V-I Measurement9/LConn2 -- Line/LConn2
  Three-Phase V-I Measurement9/LConn3 -- Line/LConn3
  " Bus13"/RConn1 -- Breaker MG/LConn1
  Transformer (T3) 4.16kV / 480 V 1 MVA/RConn3 -- Secundario 480V LL/LConn3
  Line/RConn3 -- Breaker MG/RConn3
  Primary (4.16 kV)/RConn1 -- Transformer (T3) 4.16kV / 480 V 1 MVA/LConn1
  Secundario 480V LL/RConn2 -- " Bus13"/LConn2
  Three-Phase V-I Measurement9/LConn1 -- Line/LConn1
  Primary (4.16 kV)/RConn3 -- Transformer (T3) 4.16kV / 480 V 1 MVA/LConn3
  Breaker MG1/LConn2 -- "Main Grid "/RConn2
  "Main Grid "/RConn3 -- Breaker MG1/LConn1
  "Main Grid "/RConn1 -- Breaker MG1/LConn3
  Breaker MG1/RConn3 -- Primary (4.16 kV)/LConn3
  Breaker MG1/RConn2 -- Primary (4.16 kV)/LConn2
  Breaker MG1/RConn1 -- Primary (4.16 kV)/LConn1

== system MGTestSystem_4bus/Bus_1 ==
  note: C
  note: B
  note: A
  note: C
  note: Linea - Neutro
  note: B
  note: A
  note: A
  note: B
  Conv pu1 : Gain  Gain=sqrt (3) /4.16e3  SaturateOnIntegerOverflow=on  OutDataTypeStr=Inherit: Same as input  ParamDataTypeStr=Inherit: Same as input
  Conv pu2 : Gain  Gain=sqrt (3) /4.16e3  SaturateOnIntegerOverflow=on  OutDataTypeStr=Inherit: Same as input  ParamDataTypeStr=Inherit: Same as input
  Measurement1 : Scope  NumInputPorts=4
  PLL : Subsystem
  Power Factor Block1 : Subsystem  mask(Power Factor Block){Freq=60, Vinit=[0, 0], Iinit=[0, 0], Ts=0}
      mask prompts: Freq "Fundamental frequency (Hz):"; Vinit "Voltage initial input [ Mag, Phase (degrees) ]:"; Iinit "Current initial input [ Mag, Phase (degrees) ]:"; Ts "Sample time:"
      mask help:
      | Power Factor Block developed by Dr Rodney Tan
      | Version 1.01 (Aug 2016)
      |
      | Compute power factor and phase angle of AC circuit voltage-current pair at fundamental frequency.
      |
      | The computation is based on Power block and Complex number function block.
      |
      | For the first cycle of simulation, the outputs are held constant to the powers computed for the Voltage initial input and Current initial input parameters.
      mask Help:
      | <b>Fundamental Frequency (Hz)</b>
      | Specify the measurement fundamental frequency, in hertz, of the input signal.
      | 
      | <b>Voltage initial input [ Mag, Phase (degrees) ]</b>
      | Specify the voltage initial magnitude and phase to set a constant output for the first cycle of simulation.
      | 
      | <b>Current initial input [ Mag, Phase (degrees) ]</b>
      | Specify the current initial magnitude and phase to set a constant output for the first cycle of simulation.
      | 
      | <b>Sample Time</b>
      | Specify the sample time of the block, in seconds. Set to 0 to implement a continuous block.
      mask TypeOptions Freq: Power/Freq
      mask TypeOptions Vinit: Power/Vinit
      mask TypeOptions Iinit: Power/Iinit
      mask TypeOptions Ts: Power/Ts
  Power Factor1 : Display
  Scope : Scope
  THD : spsTHDLib/THD  Freq=60  Ts=Ts_Simulation
      settings: SourceProductBaseCode=PS
  THD (% and signal) : Scope  NumInputPorts=2
  THD (%) : Display
      settings: Format=bank
  Vabc pu1 : Scope
  to % : Gain  Gain=100  SampleTime=Ts_Simulation
  ángulo de V (%)1 : Display
      settings: Format=bank
  tag scope: PFabc_Bus2=global, THDv_abc_Bus2=global, delta_abc_Bus2=global
  wires:
  [Iabc_LL_Bus2] -> Power Factor Block1/2(Iabc)
  THD/1 -> to %/1
  Power Factor Block1/4(Iabc y Iabc (rms)) -> Measurement1/4
  Power Factor Block1/1(Pabc) -> Measurement1/1
  Conv pu1/1 -> Vabc pu1/1
  Power Factor Block1/2(Qabc) -> Measurement1/2
  Power Factor Block1/3(Vabc y Vabc (rms)) -> Conv pu1/1, Measurement1/3
  to %/1 -> [THDv_abc_Bus2], THD (%)/1, THD (% and signal)/2  "THD (%)"
  Power Factor Block1/5("PFabc ") -> [PFabc_Bus2], Power Factor1/1
  PLL/1(delta_abc) -> [delta_abc_Bus2], Scope/1, ángulo de V (%)1/1
  [Vabc_LL_Bus2] -> Conv pu2/1, THD/1, THD (% and signal)/1, Power Factor Block1/1(Vabc)  "Signal Vabc"
  Conv pu2/1 -> PLL/1(Vabc_LN_pu)

== system MGTestSystem_4bus/Bus_2 ==
  note: B
  note: A
  note: A
  note: B
  note: Linea - Neutro
  note: C
  note: A
  note: B
  note: C
  Conv pu1 : Gain  Gain=sqrt (3) /4.16e3  SaturateOnIntegerOverflow=on  OutDataTypeStr=Inherit: Same as input  ParamDataTypeStr=Inherit: Same as input
  Conv pu2 : Gain  Gain=sqrt (3) /4.16e3  SaturateOnIntegerOverflow=on  OutDataTypeStr=Inherit: Same as input  ParamDataTypeStr=Inherit: Same as input
  Measurement1 : Scope  NumInputPorts=4
  PLL : Subsystem
  Power Factor Block1 : Subsystem  mask(Power Factor Block){Freq=60, Vinit=[0, 0], Iinit=[0, 0], Ts=0}
      mask prompts: Freq "Fundamental frequency (Hz):"; Vinit "Voltage initial input [ Mag, Phase (degrees) ]:"; Iinit "Current initial input [ Mag, Phase (degrees) ]:"; Ts "Sample time:"
      mask help:
      | Power Factor Block developed by Dr Rodney Tan
      | Version 1.01 (Aug 2016)
      |
      | Compute power factor and phase angle of AC circuit voltage-current pair at fundamental frequency.
      |
      | The computation is based on Power block and Complex number function block.
      |
      | For the first cycle of simulation, the outputs are held constant to the powers computed for the Voltage initial input and Current initial input parameters.
      mask Help:
      | <b>Fundamental Frequency (Hz)</b>
      | Specify the measurement fundamental frequency, in hertz, of the input signal.
      | 
      | <b>Voltage initial input [ Mag, Phase (degrees) ]</b>
      | Specify the voltage initial magnitude and phase to set a constant output for the first cycle of simulation.
      | 
      | <b>Current initial input [ Mag, Phase (degrees) ]</b>
      | Specify the current initial magnitude and phase to set a constant output for the first cycle of simulation.
      | 
      | <b>Sample Time</b>
      | Specify the sample time of the block, in seconds. Set to 0 to implement a continuous block.
      mask TypeOptions Freq: Power/Freq
      mask TypeOptions Vinit: Power/Vinit
      mask TypeOptions Iinit: Power/Iinit
      mask TypeOptions Ts: Power/Ts
  Power Factor1 : Display
  Scope : Scope
  THD : spsTHDLib/THD  Freq=60  Ts=Ts_Simulation
      settings: SourceProductBaseCode=PS
  THD (% and signal) : Scope  NumInputPorts=2
  THD (%) : Display
      settings: Format=bank
  Vabc pu1 : Scope
  to % : Gain  Gain=100  SampleTime=Ts_Simulation
  ángulo de V (%)1 : Display
      settings: Format=bank
  tag scope: PFabc_Bus1=global, THDv_abc_Bus1=global, delta_abc_Bus1=global
  wires:
  Conv pu2/1 -> PLL/1(Vabc_LN_pu)
  [Vabc_LL_Bus1] -> Power Factor Block1/1(Vabc), THD (% and signal)/1, THD/1, Conv pu2/1  "Signal Vabc"
  PLL/1(delta_abc) -> ángulo de V (%)1/1, Scope/1, [delta_abc_Bus1]
  Power Factor Block1/5("PFabc ") -> Power Factor1/1, [PFabc_Bus1]
  to %/1 -> THD (% and signal)/2, THD (%)/1, [THDv_abc_Bus1]  "THD (%)"
  Power Factor Block1/3(Vabc y Vabc (rms)) -> Measurement1/3, Conv pu1/1
  Power Factor Block1/2(Qabc) -> Measurement1/2
  Conv pu1/1 -> Vabc pu1/1
  Power Factor Block1/1(Pabc) -> Measurement1/1
  Power Factor Block1/4(Iabc y Iabc (rms)) -> Measurement1/4
  THD/1 -> to %/1
  [Iabc_LL_Bus1] -> Power Factor Block1/2(Iabc)

== system MGTestSystem_4bus/Bus_3 ==
  note: B
  note: A
  note: A
  note: B
  note: Linea - Neutro
  note: C
  note: A
  note: B
  note: C
  Conv pu1 : Gain  Gain=sqrt (3) /4.16e3  SaturateOnIntegerOverflow=on  OutDataTypeStr=Inherit: Same as input  ParamDataTypeStr=Inherit: Same as input
  Conv pu2 : Gain  Gain=sqrt (3) /4.16e3  SaturateOnIntegerOverflow=on  OutDataTypeStr=Inherit: Same as input  ParamDataTypeStr=Inherit: Same as input
  Measurement1 : Scope  NumInputPorts=4
  PLL : Subsystem
  Power Factor Block1 : Subsystem  mask(Power Factor Block){Freq=60, Vinit=[0, 0], Iinit=[0, 0], Ts=0}
      mask prompts: Freq "Fundamental frequency (Hz):"; Vinit "Voltage initial input [ Mag, Phase (degrees) ]:"; Iinit "Current initial input [ Mag, Phase (degrees) ]:"; Ts "Sample time:"
      mask help:
      | Power Factor Block developed by Dr Rodney Tan
      | Version 1.01 (Aug 2016)
      |
      | Compute power factor and phase angle of AC circuit voltage-current pair at fundamental frequency.
      |
      | The computation is based on Power block and Complex number function block.
      |
      | For the first cycle of simulation, the outputs are held constant to the powers computed for the Voltage initial input and Current initial input parameters.
      mask Help:
      | <b>Fundamental Frequency (Hz)</b>
      | Specify the measurement fundamental frequency, in hertz, of the input signal.
      | 
      | <b>Voltage initial input [ Mag, Phase (degrees) ]</b>
      | Specify the voltage initial magnitude and phase to set a constant output for the first cycle of simulation.
      | 
      | <b>Current initial input [ Mag, Phase (degrees) ]</b>
      | Specify the current initial magnitude and phase to set a constant output for the first cycle of simulation.
      | 
      | <b>Sample Time</b>
      | Specify the sample time of the block, in seconds. Set to 0 to implement a continuous block.
      mask TypeOptions Freq: Power/Freq
      mask TypeOptions Vinit: Power/Vinit
      mask TypeOptions Iinit: Power/Iinit
      mask TypeOptions Ts: Power/Ts
  Power Factor1 : Display
  Scope : Scope
  THD : spsTHDLib/THD  Freq=60  Ts=Ts_Simulation
      settings: SourceProductBaseCode=PS
  THD (% and signal) : Scope  NumInputPorts=2
  THD (%) : Display
      settings: Format=bank
  Vabc pu1 : Scope
  to % : Gain  Gain=100  SampleTime=Ts_Simulation
  ángulo de V (%)1 : Display
      settings: Format=bank
  tag scope: PFabc_Bus3=global, THDv_abc_Bus3=global, delta_abc_Bus3=global
  wires:
  Conv pu2/1 -> PLL/1(Vabc_LN_pu)
  [Vabc_LL_Bus3] -> Power Factor Block1/1(Vabc), THD (% and signal)/1, THD/1, Conv pu2/1  "Signal Vabc"
  PLL/1(delta_abc) -> ángulo de V (%)1/1, Scope/1, [delta_abc_Bus3]
  Power Factor Block1/5("PFabc ") -> Power Factor1/1, [PFabc_Bus3]
  to %/1 -> THD (% and signal)/2, THD (%)/1, [THDv_abc_Bus3]  "THD (%)"
  Power Factor Block1/3(Vabc y Vabc (rms)) -> Measurement1/3, Conv pu1/1
  Power Factor Block1/2(Qabc) -> Measurement1/2
  Conv pu1/1 -> Vabc pu1/1
  Power Factor Block1/1(Pabc) -> Measurement1/1
  Power Factor Block1/4(Iabc y Iabc (rms)) -> Measurement1/4
  THD/1 -> to %/1
  [Iabc_LL_Bus3] -> Power Factor Block1/2(Iabc)

== system MGTestSystem_4bus/Bus_4 ==
  note: C
  note: B
  note: A
  note: C
  note: Linea - Neutro
  note: B
  note: A
  note: A
  note: B
  Conv pu1 : Gain  Gain=sqrt (3) /4.16e3  SaturateOnIntegerOverflow=on  OutDataTypeStr=Inherit: Same as input  ParamDataTypeStr=Inherit: Same as input
  Conv pu2 : Gain  Gain=sqrt (3) /4.16e3  SaturateOnIntegerOverflow=on  OutDataTypeStr=Inherit: Same as input  ParamDataTypeStr=Inherit: Same as input
  Measurement1 : Scope  NumInputPorts=4
  PLL : Subsystem
  Power Factor Block1 : Subsystem  mask(Power Factor Block){Freq=60, Vinit=[0, 0], Iinit=[0, 0], Ts=0}
      mask prompts: Freq "Fundamental frequency (Hz):"; Vinit "Voltage initial input [ Mag, Phase (degrees) ]:"; Iinit "Current initial input [ Mag, Phase (degrees) ]:"; Ts "Sample time:"
      mask help:
      | Power Factor Block developed by Dr Rodney Tan
      | Version 1.01 (Aug 2016)
      |
      | Compute power factor and phase angle of AC circuit voltage-current pair at fundamental frequency.
      |
      | The computation is based on Power block and Complex number function block.
      |
      | For the first cycle of simulation, the outputs are held constant to the powers computed for the Voltage initial input and Current initial input parameters.
      mask Help:
      | <b>Fundamental Frequency (Hz)</b>
      | Specify the measurement fundamental frequency, in hertz, of the input signal.
      | 
      | <b>Voltage initial input [ Mag, Phase (degrees) ]</b>
      | Specify the voltage initial magnitude and phase to set a constant output for the first cycle of simulation.
      | 
      | <b>Current initial input [ Mag, Phase (degrees) ]</b>
      | Specify the current initial magnitude and phase to set a constant output for the first cycle of simulation.
      | 
      | <b>Sample Time</b>
      | Specify the sample time of the block, in seconds. Set to 0 to implement a continuous block.
      mask TypeOptions Freq: Power/Freq
      mask TypeOptions Vinit: Power/Vinit
      mask TypeOptions Iinit: Power/Iinit
      mask TypeOptions Ts: Power/Ts
  Power Factor1 : Display
  Scope : Scope
  THD : spsTHDLib/THD  Freq=60  Ts=Ts_Simulation
      settings: SourceProductBaseCode=PS
  THD (% and signal) : Scope  NumInputPorts=2
  THD (%) : Display
      settings: Format=bank
  Vabc pu1 : Scope
  to % : Gain  Gain=100  SampleTime=Ts_Simulation
  ángulo de V (%)1 : Display
      settings: Format=bank
  tag scope: PFabc_Bus4=global, THDv_abc_Bus4=global, delta_abc_Bus4=global
  wires:
  [Iabc_LL_Bus4] -> Power Factor Block1/2(Iabc)
  THD/1 -> to %/1
  Power Factor Block1/4(Iabc y Iabc (rms)) -> Measurement1/4
  Power Factor Block1/1(Pabc) -> Measurement1/1
  Conv pu1/1 -> Vabc pu1/1
  Power Factor Block1/2(Qabc) -> Measurement1/2
  Power Factor Block1/3(Vabc y Vabc (rms)) -> Conv pu1/1, Measurement1/3
  to %/1 -> [THDv_abc_Bus4], THD (%)/1, THD (% and signal)/2  "THD (%)"
  Power Factor Block1/5("PFabc ") -> [PFabc_Bus4], Power Factor1/1
  PLL/1(delta_abc) -> [delta_abc_Bus4], Scope/1, ángulo de V (%)1/1
  [Vabc_LL_Bus4] -> Conv pu2/1, THD/1, THD (% and signal)/1, Power Factor Block1/1(Vabc)  "Signal Vabc"
  Conv pu2/1 -> PLL/1(Vabc_LN_pu)

== system MGTestSystem_4bus/Bus_6 ==
  note: C
  note: B
  note: A
  note: C
  note: Linea - Neutro
  note: B
  note: A
  note: A
  note: B
  Conv pu1 : Gain  Gain=sqrt (3) /4.16e3  SaturateOnIntegerOverflow=on  OutDataTypeStr=Inherit: Same as input  ParamDataTypeStr=Inherit: Same as input
  Conv pu2 : Gain  Gain=sqrt (3) /4.16e3  SaturateOnIntegerOverflow=on  OutDataTypeStr=Inherit: Same as input  ParamDataTypeStr=Inherit: Same as input
  Measurement1 : Scope  NumInputPorts=4
  PLL : Subsystem
  Power Factor Block1 : Subsystem  mask(Power Factor Block){Freq=60, Vinit=[0, 0], Iinit=[0, 0], Ts=0}
      mask prompts: Freq "Fundamental frequency (Hz):"; Vinit "Voltage initial input [ Mag, Phase (degrees) ]:"; Iinit "Current initial input [ Mag, Phase (degrees) ]:"; Ts "Sample time:"
      mask help:
      | Power Factor Block developed by Dr Rodney Tan
      | Version 1.01 (Aug 2016)
      |
      | Compute power factor and phase angle of AC circuit voltage-current pair at fundamental frequency.
      |
      | The computation is based on Power block and Complex number function block.
      |
      | For the first cycle of simulation, the outputs are held constant to the powers computed for the Voltage initial input and Current initial input parameters.
      mask Help:
      | <b>Fundamental Frequency (Hz)</b>
      | Specify the measurement fundamental frequency, in hertz, of the input signal.
      | 
      | <b>Voltage initial input [ Mag, Phase (degrees) ]</b>
      | Specify the voltage initial magnitude and phase to set a constant output for the first cycle of simulation.
      | 
      | <b>Current initial input [ Mag, Phase (degrees) ]</b>
      | Specify the current initial magnitude and phase to set a constant output for the first cycle of simulation.
      | 
      | <b>Sample Time</b>
      | Specify the sample time of the block, in seconds. Set to 0 to implement a continuous block.
      mask TypeOptions Freq: Power/Freq
      mask TypeOptions Vinit: Power/Vinit
      mask TypeOptions Iinit: Power/Iinit
      mask TypeOptions Ts: Power/Ts
  Power Factor1 : Display
  Scope : Scope
  THD : spsTHDLib/THD  Freq=60  Ts=Ts_Power
      settings: SourceProductBaseCode=PS
  THD (% and signal) : Scope  NumInputPorts=2
  THD (%) : Display
      settings: Format=bank
  Vabc pu1 : Scope
  to % : Gain  Gain=100  SampleTime=Ts_Power
  ángulo de V (%)1 : Display
      settings: Format=bank
  tag scope: PFabc_Bus0=global, THDv_abc_Bus0=global, delta_abc_Bus0=global
  wires:
  [Iabc_LL_Bus13] -> Power Factor Block1/2(Iabc)
  THD/1 -> to %/1
  Power Factor Block1/4(Iabc y Iabc (rms)) -> Measurement1/4
  Power Factor Block1/1(Pabc) -> Measurement1/1
  Conv pu1/1 -> Vabc pu1/1
  Power Factor Block1/2(Qabc) -> Measurement1/2
  Power Factor Block1/3(Vabc y Vabc (rms)) -> Conv pu1/1, Measurement1/3
  to %/1 -> THD (%)/1, [THDv_abc_Bus0], THD (% and signal)/2  "THD (%)"
  Power Factor Block1/5("PFabc ") -> Power Factor1/1, [PFabc_Bus0]
  PLL/1(delta_abc) -> [delta_abc_Bus0], Scope/1, ángulo de V (%)1/1
  [Vabc_LL_Bus13] -> Conv pu2/1, THD/1, THD (% and signal)/1, Power Factor Block1/1(Vabc)  "Signal Vabc"
  Conv pu2/1 -> PLL/1(Vabc_LN_pu)

== system MGTestSystem_4bus/DATA  ADQUISITION ==
  Delta_abc : Subsystem
  Measured data (PMU) : Subsystem
  PF_abc : Subsystem
  P_abc : Subsystem
  Power_Losses_abc : Subsystem  Commented=on
  Q_abc : Subsystem
  THDv_abc : Subsystem
  VoltageLL_pu_abc : Subsystem
